simulink model "DSP_Project"  (R2016a)
settings: Solver=VariableStepAuto  StartTime=0.0  StopTime=2  RelTol=1e-3
libraries: simulink x11
settings Model: Creator=100491359  LastModifiedBy=100491359

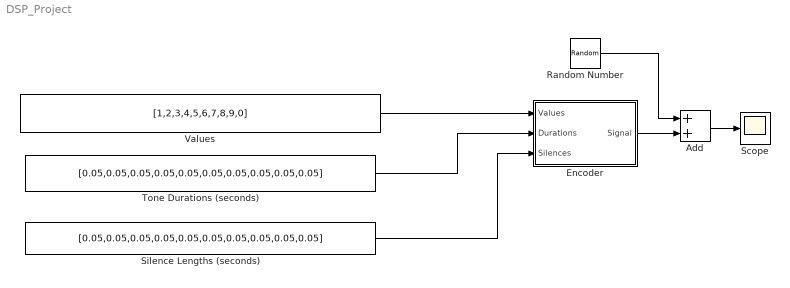
== system DSP_Project ==
  Add : Sum
  Encoder : Subsystem
  Random Number : RandomNumber  Variance=0.01  SampleTime=1/8000
  Scope : Scope
  Silence Lengths (seconds) : Constant  Value=[0.05,0.05,0.05,0.05,0.05,0.05,0.05,0.05,0.05,0.05]  VectorParams1D=off  SampleTime=1/8000
  Tone Durations (seconds) : Constant  Value=[0.05,0.05,0.05,0.05,0.05,0.05,0.05,0.05,0.05,0.05]  VectorParams1D=off  SampleTime=1/8000
  "Values " : Constant  Value=[1,2,3,4,5,6,7,8,9,0]  VectorParams1D=off  SampleTime=1/8000
  wires:
  Tone Durations (seconds)/1 -> Encoder/2(Durations)
  Silence Lengths (seconds)/1 -> Encoder/3(Silences)
  "Values "/1 -> Encoder/1(Values)
  Encoder/1(Signal) -> Add/2
  Random Number/1 -> Add/1
  Add/1 -> Scope/1

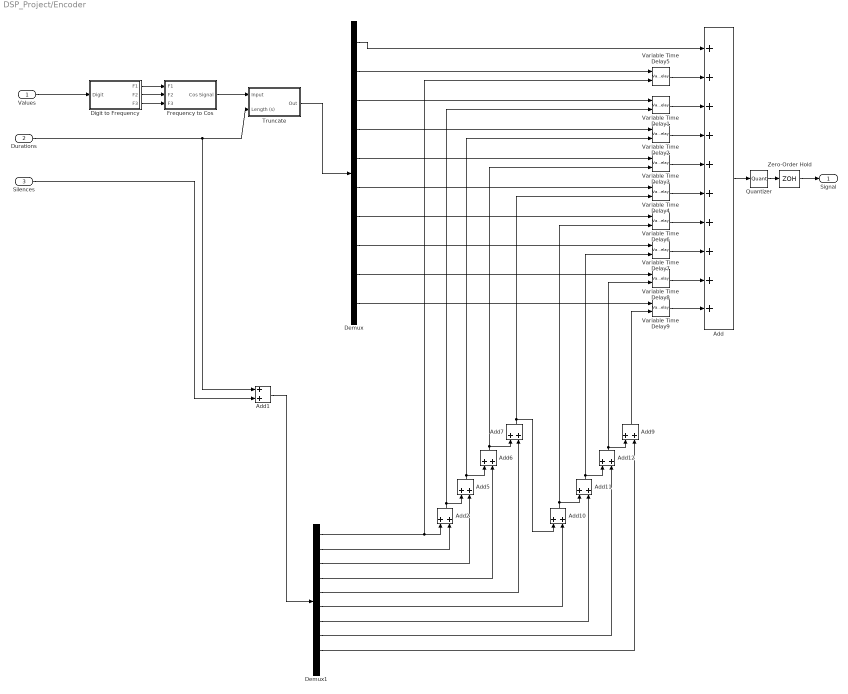
== system DSP_Project/Encoder ==
  Values : Inport
  Durations : Inport  Port=2
  Silences : Inport  Port=3
  Add : Sum  Inputs=++++++++++
  Add{1..2,5..7,9..12} (9 alike) : Sum
  Demux : Demux  Outputs=10
  Demux1 : Demux  Outputs=10
  Digit to Frequency : Subsystem
  Frequency to Cos : Subsystem
  Quantizer : Quantizer  QuantizationInterval=1/8000
  "Truncate " : Subsystem
  Variable Time Delay{1..9} (9 alike) : VariableTransportDelay  MaximumDelay=10  ZeroDelay=on
  Zero-Order Hold : ZeroOrderHold  SampleTime=1/8000
  Signal : Outport
  wires:
  Digit to Frequency/3(F3) -> Frequency to Cos/3(F3)
  Digit to Frequency/2(F2) -> Frequency to Cos/2(F2)
  Digit to Frequency/1(F1) -> Frequency to Cos/1(F1)
  Demux1/2 -> Add2/2
  Add6/1 -> Variable Time Delay3/2, Add7/1
  Demux1/7 -> Add11/2
  Add10/1 -> Variable Time Delay6/2, Add11/1
  Demux1/9 -> Add9/2
  Variable Time Delay4/1 -> Add/6
  Demux1/6 -> Add10/2
  Add7/1 -> Variable Time Delay4/2, Add10/1
  Demux/7 -> Variable Time Delay6/1
  Demux1/3 -> Add5/2
  Add9/1 -> Variable Time Delay9/2
  Variable Time Delay5/1 -> Add/2
  Values/1 -> Digit to Frequency/1("Digit ")
  Durations/1 -> "Truncate "/2(Length (s)), Add1/1
  "Truncate "/1(Out) -> Demux/1
  Frequency to Cos/1(Cos Signal) -> "Truncate "/1(Input)
  Demux1/5 -> Add7/2
  Add11/1 -> Variable Time Delay7/2, Add12/1
  Add5/1 -> Variable Time Delay2/2, Add6/1
  Demux/2 -> Variable Time Delay5/1
  Demux/4 -> Variable Time Delay2/1
  Demux/8 -> Variable Time Delay7/1
  Variable Time Delay2/1 -> Add/4
  Add1/1 -> Demux1/1
  Silences/1 -> Add1/2
  Demux1/8 -> Add12/2
  Demux/6 -> Variable Time Delay4/1
  Demux/9 -> Variable Time Delay8/1
  Add12/1 -> Add9/1, Variable Time Delay8/2
  Variable Time Delay7/1 -> Add/8
  Variable Time Delay9/1 -> Add/10
  Demux/10 -> Variable Time Delay9/1
  Demux/5 -> Variable Time Delay3/1
  Demux/1 -> Add/1
  Variable Time Delay1/1 -> Add/3
  Demux/3 -> Variable Time Delay1/1
  Variable Time Delay6/1 -> Add/7
  Variable Time Delay8/1 -> Add/9
  Variable Time Delay3/1 -> Add/5
  Demux1/4 -> Add6/2
  Demux1/1 -> Variable Time Delay5/2, Add2/1
  Add2/1 -> Variable Time Delay1/2, Add5/1
  Quantizer/1 -> Zero-Order Hold/1
  Add/1 -> Quantizer/1
  Zero-Order Hold/1 -> Signal/1

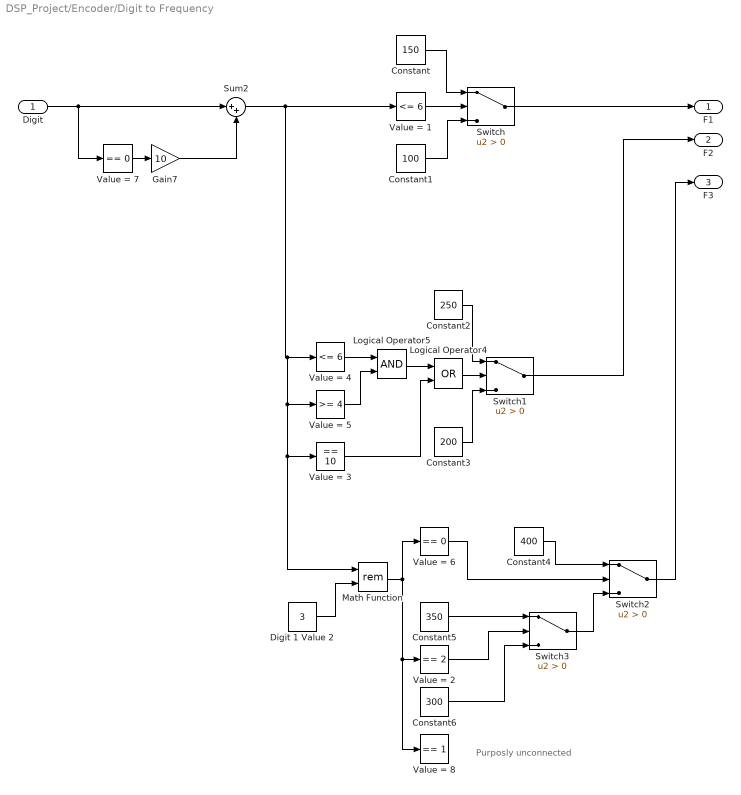
== system DSP_Project/Encoder/Digit to Frequency ==
  note: Purposly unconnected
  "Digit " : Inport
  Constant : Constant  Value=150  SampleTime=1/8000
  Constant1 : Constant  Value=100  SampleTime=1/8000
  Constant2 : Constant  Value=250  SampleTime=1/8000
  Constant3 : Constant  Value=200  SampleTime=1/8000
  Constant4 : Constant  Value=400  SampleTime=1/8000
  Constant5 : Constant  Value=350  SampleTime=1/8000
  Constant6 : Constant  Value=300  SampleTime=1/8000
  Digit 1 Value 2 : Constant  Value=3  SampleTime=1/8000
  Gain7 : Gain  Gain=10
  Logical Operator4 : Logic  Operator=OR  AllPortsSameDT=off  OutDataTypeStr=boolean
  Logical Operator5 : Logic  AllPortsSameDT=off  OutDataTypeStr=boolean
  Math Function : Math  Operator=rem  SaturateOnIntegerOverflow=on
  Sum2 : Sum  Inputs=|++
  Switch{,1..3} (4 alike) : Switch  Criteria=u2 > Threshold
  Value = 1 : simulink/Logic and Bit Operations/Compare To Constant  relop=<=  const=6  OutDataTypeStr=boolean
  Value = 2 : simulink/Logic and Bit Operations/Compare To Constant  relop===  const=2  OutDataTypeStr=boolean
  Value = 3 : simulink/Logic and Bit Operations/Compare To Constant  relop===  const=10  OutDataTypeStr=boolean
  Value = 4 : simulink/Logic and Bit Operations/Compare To Constant  relop=<=  const=6  OutDataTypeStr=boolean
  Value = 5 : simulink/Logic and Bit Operations/Compare To Constant  relop=>=  const=4  OutDataTypeStr=boolean
  Value = 6 : simulink/Logic and Bit Operations/Compare To Constant  relop===  const=0  OutDataTypeStr=boolean
  Value = 7 : simulink/Logic and Bit Operations/Compare To Constant  relop===  const=0  OutDataTypeStr=boolean
  Value = 8 : simulink/Logic and Bit Operations/Compare To Constant  relop===  const=1  OutDataTypeStr=boolean
  F1 : Outport
  F2 : Outport  Port=2
  F3 : Outport  Port=3
  wires:
  Logical Operator5/1 -> Logical Operator4/1
  Math Function/1 -> Value = 6/1, Value = 8/1, Value = 2/1
  Value = 6/1 -> Switch2/2
  Value = 4/1 -> Logical Operator5/1
  Value = 3/1 -> Logical Operator4/2
  Value = 5/1 -> Logical Operator5/2
  Digit 1 Value 2/1 -> Math Function/2
  Logical Operator4/1 -> Switch1/2
  Sum2/1 -> Math Function/1, Value = 3/1, Value = 5/1, Value = 4/1, Value = 1/1
  Gain7/1 -> Sum2/2
  "Digit "/1 -> Value = 7/1, Sum2/1
  Switch1/1 -> F2/1
  Switch/1 -> F1/1
  Value = 7/1 -> Gain7/1
  Value = 1/1 -> Switch/2
  Constant/1 -> Switch/1
  Constant1/1 -> Switch/3
  Constant2/1 -> Switch1/1
  Constant3/1 -> Switch1/3
  Constant4/1 -> Switch2/1
  Value = 2/1 -> Switch3/2
  Switch3/1 -> Switch2/3
  Constant5/1 -> Switch3/1
  Constant6/1 -> Switch3/3
  Switch2/1 -> F3/1

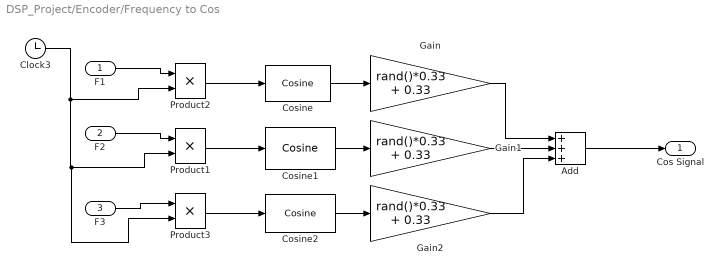
== system DSP_Project/Encoder/Frequency to Cos ==
  F1 : Inport
  F2 : Inport  Port=2
  F3 : Inport  Port=3
  Add : Sum  Inputs=+++
  Clock3 : Clock
  Cosine : simulink/Lookup Tables/Cosine  Formula=cos(2*pi*u)  NumDataPoints=(2^5)+1  OutputWordLength=16  InternalRulePriority=Speed
  Cosine1 : simulink/Lookup Tables/Cosine  Formula=cos(2*pi*u)  NumDataPoints=(2^5)+1  OutputWordLength=16  InternalRulePriority=Speed
  Cosine2 : simulink/Lookup Tables/Cosine  Formula=cos(2*pi*u)  NumDataPoints=(2^5)+1  OutputWordLength=16  InternalRulePriority=Speed
  Gain : Gain  Gain=rand()*0.33 + 0.33
  Gain1 : Gain  Gain=rand()*0.33 + 0.33
  Gain2 : Gain  Gain=rand()*0.33 + 0.33
  Product1 : Product
  Product2 : Product
  Product3 : Product
  Cos Signal : Outport
  wires:
  Product2/1 -> Cosine/1
  Product1/1 -> Cosine1/1
  Product3/1 -> Cosine2/1
  F2/1 -> Product1/1
  Clock3/1 -> Product2/2, Product3/2, Product1/2
  F1/1 -> Product2/1
  F3/1 -> Product3/1
  Gain/1 -> Add/1
  Gain1/1 -> Add/2
  Gain2/1 -> Add/3
  Add/1 -> Cos Signal/1
  Cosine2/1 -> Gain2/1
  Cosine1/1 -> Gain1/1
  Cosine/1 -> Gain/1

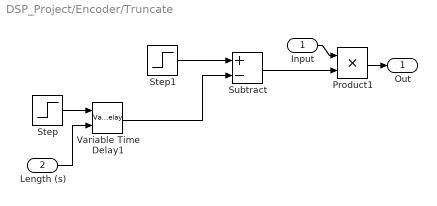
== system DSP_Project/Encoder/Truncate  ==
  Input : Inport
  Length (s) : Inport  Port=2
  Product1 : Product
  Step : Step  Time=0  SampleTime=1/8000
  Step1 : Step  Time=0  SampleTime=1/8000
  Subtract : Sum  Inputs=+-
  Variable Time Delay1 : VariableTransportDelay  MaximumDelay=10  ZeroDelay=on
  Out : Outport
  wires:
  Subtract/1 -> Product1/2
  Variable Time Delay1/1 -> Subtract/2
  Step/1 -> Variable Time Delay1/1
  Step1/1 -> Subtract/1
  Input/1 -> Product1/1
  Product1/1 -> Out/1
  Length (s)/1 -> Variable Time Delay1/2
